simulink model "draft7"  (R2023a)
settings: Solver=VariableStepAuto  StartTime=0.0  StopTime=10  FixedStep=0.0001  MaxStep=0.1  RelTol=1e-3  AbsTol=1e-3  EnableMultiTasking=on
model workspace (MAT data in the model file):
  C_Gimbal = 0.1
  C_IAP = 0.01
  IAP_Pa = 0
  K_Gimbal = 0
  K_IAP = 10
  LeftAbdominalMuscleForce = 0
  LeftBackMuscleForce = 0
  LeftTransverse1MuscleForce = 0
  LeftTransverse2MuscleForce = 0
  Moment_AR = 0
  Moment_FE = 0
  Moment_LB = 0
  RightAbdominalMuscleForce = 0
  RightBackMuscleForce = 0
  RightTransverse1MuscleForce = 0
  RightTransverse2MuscleForce = 0
  a = 1
  b = 1
undefined symbols (not defined in the file): X, Y, Z
libraries: sm_lib x279, nesl_utility x233, simulink_extras x33, checkpacklib x3, simulink x1
(part 6 of 7)

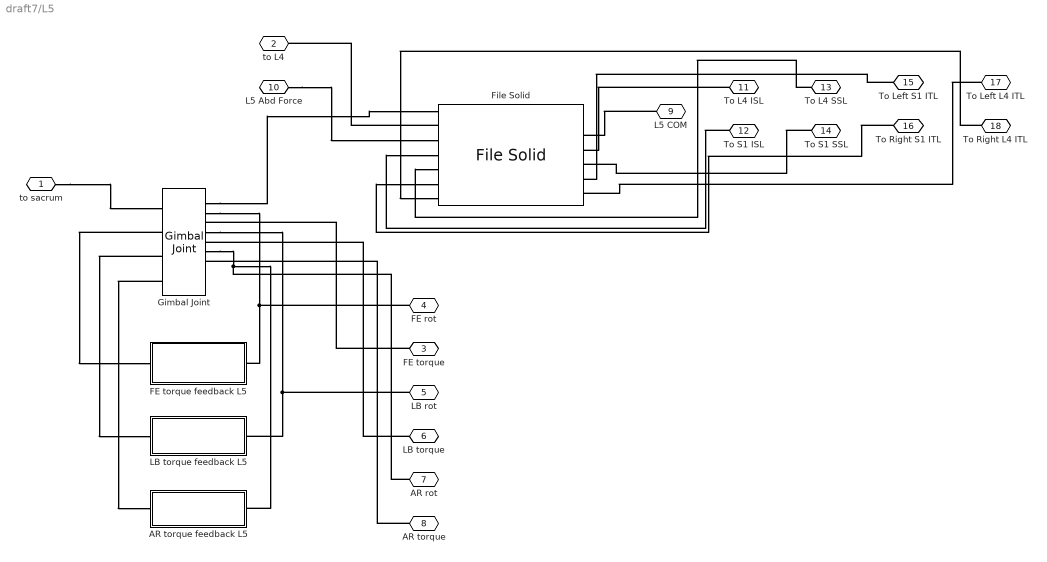
== system draft7/L5 ==
  AR torque feedback L5 : Subsystem
  FE torque feedback L5 : Subsystem
  File Solid : sm_lib/Body Elements/File Solid  ExtGeomFileName=C:\Users\siril\OneDrive\Desktop\TIM-Control\Matlab\Simscape models\CAD - with COM\SymmetricModel\draft7\L5.step  UnitType=FromFile  ExtGeomFileUnits=m  StepReaderType=HEX  ExportConvexHullGeometry=off  InertiaType=CalculateFromGeometry  Mass=1  MassUnits=kg  CenterOfMass=[0 0 0]  CenterOfMassUnits=m  MomentsOfInertia=[1 1 1]  MomentsOfInertiaUnits=kg*m^2  ProductsOfInertia=[0 0 0]  ProductsOfInertiaUnits=kg*m^2  BasedOnType=Density  Density=0.182  DensityUnits=g/cm^3  DoExposeReferenceFrame=on  SerializedFrames=<Frames><Frame><Id>Frame1</Id><Value><Name>To Sacrum</Name><Origin><Source>GeometricFeature</Source><FeatureName>planar surface 1973</FeatureName></Origin><PrimaryAxis><DefinedDirection>+Z</DefinedDirection><Source>GeometricFeature</Source><SourceDirection>+Z</SourceDirection><FeatureName>planar surface 1973</FeatureName></PrimaryAxis><SecondaryAxis><DefinedDirection>+X</DefinedDirection><Source>ReferenceFrame</Source><SourceDirection>+X</SourceDirection><FeatureName></FeatureName></SecondaryAxis></Value></Frame><Frame><Id>Frame2</Id><Value><Name>To L4</Name><Origin><Source>GeometricFeature</Source><FeatureName>planar surface 1977</FeatureName></Origin><PrimaryAxis><DefinedDirection>+Z</DefinedDirection><Source>GeometricFeature</Source><SourceDirection>+Z</SourceDirection><FeatureName>planar surface 1977</FeatureName></PrimaryAxis><SecondaryAxis><DefinedDirection>+X</DefinedDirection><Source>ReferenceFrame</Source><SourceDirection>+X</SourceDirection><FeatureName></FeatureName></SecondaryAxis></Value></Frame><Frame><Id>Frame3</Id><Value><Name>L5 COM</Name><Origin><Source>CenterOfMassFrame</Source><FeatureName></FeatureName></Origin><PrimaryAxis><DefinedDirection>+Z</DefinedDirection><Source>ReferenceFrame</Source><SourceDirection>+Z</SourceDirection><FeatureName></FeatureName></PrimaryAxis><SecondaryAxis><DefinedDirection>+X</DefinedDirection><Source>ReferenceFrame</Source><SourceDirection>+X</SourceDirection><FeatureName></FeatureName></SecondaryAxis></Value></Frame><Frame><Id>Frame4</Id><Value><Name>L5 Abd Force</Name><Origin><Source>GeometricFeature</Source><FeatureName>point 2</FeatureName></Origin><PrimaryAxis><DefinedDirection>+Z</DefinedDirection><Source>GeometricFeature</Source><SourceDirection>+Z</SourceDirection><FeatureName>conical surface 1</FeatureName></PrimaryAxis><SecondaryAxis><DefinedDirection>+X</DefinedDirection><Source>ReferenceFrame</Source><SourceDirection>+X</SourceDirection><FeatureName></FeatureName></SecondaryAxis></Value></Frame><Frame><Id>Frame5</Id><Value><Name>To L4 ISL</Name><Origin><Source>GeometricFeature</Source><FeatureName>point 104</FeatureName></Origin><PrimaryAxis><DefinedDirection>+Z</DefinedDirection><Source>ReferenceFrame</Source><SourceDirection>+Z</SourceDirection><FeatureName></FeatureName></PrimaryAxis><SecondaryAxis><DefinedDirection>+X</DefinedDirection><Source>ReferenceFrame</Source><SourceDirection>+X</SourceDirection><FeatureName></FeatureName></SecondaryAxis></Value></Frame><Frame><Id>Frame6</Id><Value><Name>To S1 ISL</Name><Origin><Source>GeometricFeature</Source><FeatureName>point 11405</FeatureName></Origin><PrimaryAxis><DefinedDirection>+Z</DefinedDirection><Source>ReferenceFrame</Source><SourceDirection>+Z</SourceDirection><FeatureName></FeatureName></PrimaryAxis><SecondaryAxis><DefinedDirection>+X</DefinedDirection><Source>ReferenceFrame</Source><SourceDirection>+X</SourceDirection><FeatureName></FeatureName></SecondaryAxis></Value></Frame><Frame><Id>Frame7</Id><Value><Name>To S1 SSL</Name><Origin><Source>GeometricFeature</Source><FeatureName>point 8728</FeatureName></Origin><PrimaryAxis><DefinedDirection>+Z</DefinedDirection><Source>ReferenceFrame</Source><SourceDirection>+Z</SourceDirection><FeatureName></FeatureName></PrimaryAxis><SecondaryAxis><DefinedDirection>+X</DefinedDirection><Source>ReferenceFrame</Source><SourceDirection>+X</SourceDirection><FeatureName></FeatureName></SecondaryAxis></Value></Frame><Frame><Id>Frame8</Id><Value><Name>To L4 SSL</Name><Origin><Source>GeometricFeature</Source><FeatureName>point 5958</FeatureName></Origin><PrimaryAxis><DefinedDirection>+Z</DefinedDirection><Source>ReferenceFrame</Source><SourceDirection>+Z</SourceDirection><FeatureName></FeatureName></PrimaryAxis><SecondaryAxis><DefinedDirection>+X</DefinedDirection><Source>ReferenceFrame</Source><SourceDirection>+X</SourceDirection><FeatureName></FeatureName></SecondaryAxis></Value></Frame><Frame><Id>Frame9</Id><Value><Name>To Left S1 ITL</Name><Origin><Source>GeometricFeature</Source><FeatureName>point 9071</FeatureName></Origin><PrimaryAxis><DefinedDirection>+Z</DefinedDirection><Source>ReferenceFrame</Source><SourceDirection>+Z</SourceDirection><FeatureName></FeatureName></PrimaryAxis><SecondaryAxis><DefinedDirection>+X</DefinedDirection><Source>ReferenceFrame</Source><SourceDirection>+X</SourceDirection><FeatureName></FeatureName></SecondaryAxis></Value></Frame><Frame><Id>Frame10</Id><Value><Name>To Right S1 ITL</Name><Origin><Source>GeometricFeature</Source><FeatureName>point 3312</FeatureName></Origin><PrimaryAxis><DefinedDirection>+Z</DefinedDirection><Source>ReferenceFrame</Source><SourceDirection>+Z</SourceDirection><FeatureName></FeatureName></PrimaryAxis><SecondaryAxis><DefinedDirection>+X</DefinedDirection><Source>ReferenceFrame</Source><SourceDirection>+X</SourceDirection><FeatureName></FeatureName></SecondaryAxis></Value></Frame><Frame><Id>Frame11</Id><Value><Name>To Left L4 ITL</Name><Origin><Source>GeometricFeature</Source><FeatureName>point 10699</FeatureName></Origin><PrimaryAxis><DefinedDirection>+Z</DefinedDirection><Source>ReferenceFrame</Source><SourceDirection>+Z</SourceDirection><FeatureName></FeatureName></PrimaryAxis><SecondaryAxis><DefinedDirection>+X</DefinedDirection><Source>ReferenceFrame</Source><SourceDirection>+X</SourceDirection><FeatureName></FeatureName></SecondaryAxis></Value></Frame><Frame><Id>Frame12</Id><Value><Name>To Right L4 ITL</Name><Origin><Source>GeometricFeature</Source><FeatureName>point 5014</FeatureName></Origin><PrimaryAxis><DefinedDirection>+Z</DefinedDirection><Source>ReferenceFrame</Source><SourceDirection>+Z</SourceDirection><FeatureName></FeatureName></PrimaryAxis><SecondaryAxis><DefinedDirection>+X</DefinedDirection><Source>ReferenceFrame</Source><SourceDirection>+X</SourceDirection><FeatureName></FeatureName></SecondaryAxis></Value></Frame></Frames>  GraphicType=FromGeometry  MarkerShape=Sphere  MarkerSize=10  GraphicVisPropType=SimpleVisualProperties  GraphicDiffuseColor=[0.5 0.5 0.5]  GraphicSpecularColor=[0.5 0.5 0.5 1.0]  GraphicAmbientColor=[0.15 0.15 0.15 1.0]  GraphicEmissiveColor=[0.0 0.0 0.0 1.0]  GraphicShininess=75  GraphicOpacity=1.0
  Gimbal Joint : sm_lib/Joints/Gimbal Joint  JointMode=Normal  SenseConstraintForce=on  SenseConstraintForceX=off  SenseConstraintForceY=off  SenseConstraintForceZ=off  SenseConstraintTorque=off  SenseConstraintTorqueX=off  SenseConstraintTorqueY=off  SenseConstraintTorqueZ=off  SenseTotalForce=on  SenseTotalForceX=off  SenseTotalForceY=off  SenseTotalForceZ=off  SenseTotalTorque=off  SenseTotalTorqueX=off  SenseTotalTorqueY=off  SenseTotalTorqueZ=off  CompositeWrenchDir=FollowerOnBase  CompositeWrenchFrame=BaseFrame  RxEquilibriumPosition=0  RxEquilibriumPositionUnits=deg  RxSpringStiffness=K_Gimbal  RxSpringStiffnessUnits=N*m/deg  RxDampingCoefficient=C_Gimbal  RxDampingCoefficientUnits=N*m/(deg/s)  RxTorqueActuationMode=InputTorque  RxMotionActuationMode=ComputedMotion  RxSensePosition=on  RxSenseVelocity=off  RxSenseAcceleration=off  RxSenseTorqueForce=on  RxSenseLowerLimitTorqueForce=off  RxSenseUpperLimitTorqueForce=off  RxLowerLimitSpecify=on  RxLowerLimitBound=-30  RxLowerLimitBoundUnits=deg  RxLowerLimitStiffness=10000  RxLowerLimitStiffnessUnits=N*m/deg  RxLowerLimitDamping=100  RxLowerLimitDampingUnits=N*m/(deg/s)  RxLowerLimitTransitionRegionWidth=0.1  RxLowerLimitTransitionRegionWidthUnits=deg  RxUpperLimitSpecify=on  RxUpperLimitBound=30  RxUpperLimitBoundUnits=deg  RxUpperLimitStiffness=10000  RxUpperLimitStiffnessUnits=N*m/deg  RxUpperLimitDamping=100  RxUpperLimitDampingUnits=N*m/(deg/s)  RxUpperLimitTransitionRegionWidth=0.1  RxUpperLimitTransitionRegionWidthUnits=deg  RxPositionTargetSpecify=off  RxPositionTargetPriority=High  RxPositionTargetValue=0  RxPositionTargetValueUnits=deg  RxVelocityTargetSpecify=off  RxVelocityTargetPriority=High  RxVelocityTargetValue=0  RxVelocityTargetValueUnits=deg/s  RyEquilibriumPosition=0  RyEquilibriumPositionUnits=deg  RySpringStiffness=K_Gimbal  RySpringStiffnessUnits=N*m/deg  RyDampingCoefficient=C_Gimbal  RyDampingCoefficientUnits=N*m/(deg/s)  RyTorqueActuationMode=InputTorque  RyMotionActuationMode=ComputedMotion  RySensePosition=on  RySenseVelocity=off  RySenseAcceleration=off  RySenseTorqueForce=on  RySenseLowerLimitTorqueForce=off  RySenseUpperLimitTorqueForce=off  RyLowerLimitSpecify=on  RyLowerLimitBound=-30  RyLowerLimitBoundUnits=deg  RyLowerLimitStiffness=10000  RyLowerLimitStiffnessUnits=N*m/deg  RyLowerLimitDamping=100  RyLowerLimitDampingUnits=N*m/(deg/s)  RyLowerLimitTransitionRegionWidth=0.1  RyLowerLimitTransitionRegionWidthUnits=deg  RyUpperLimitSpecify=on  RyUpperLimitBound=30  RyUpperLimitBoundUnits=deg  RyUpperLimitStiffness=10000  RyUpperLimitStiffnessUnits=N*m/deg  RyUpperLimitDamping=100  RyUpperLimitDampingUnits=N*m/(deg/s)  RyUpperLimitTransitionRegionWidth=0.1  RyUpperLimitTransitionRegionWidthUnits=deg  RyPositionTargetSpecify=off  RyPositionTargetPriority=High  RyPositionTargetValue=0  RyPositionTargetValueUnits=deg  RyVelocityTargetSpecify=off  RyVelocityTargetPriority=High  RyVelocityTargetValue=0  RyVelocityTargetValueUnits=deg/s  RzEquilibriumPosition=0  RzEquilibriumPositionUnits=deg  RzSpringStiffness=K_Gimbal  RzSpringStiffnessUnits=N*m/deg  RzDampingCoefficient=C_Gimbal  RzDampingCoefficientUnits=N*m/(deg/s)  RzTorqueActuationMode=InputTorque  RzMotionActuationMode=ComputedMotion  RzSensePosition=on  RzSenseVelocity=off  RzSenseAcceleration=off  RzSenseTorqueForce=on  RzSenseLowerLimitTorqueForce=off  RzSenseUpperLimitTorqueForce=off  RzLowerLimitSpecify=on  RzLowerLimitBound=-30  RzLowerLimitBoundUnits=deg  RzLowerLimitStiffness=10000  RzLowerLimitStiffnessUnits=N*m/deg  RzLowerLimitDamping=100  RzLowerLimitDampingUnits=N*m/(deg/s)  RzLowerLimitTransitionRegionWidth=0.1  RzLowerLimitTransitionRegionWidthUnits=deg  RzUpperLimitSpecify=on  RzUpperLimitBound=30  RzUpperLimitBoundUnits=deg  RzUpperLimitStiffness=10000  RzUpperLimitStiffnessUnits=N*m/deg  RzUpperLimitDamping=100  RzUpperLimitDampingUnits=N*m/(deg/s)  RzUpperLimitTransitionRegionWidth=0.1  RzUpperLimitTransitionRegionWidthUnits=deg  RzPositionTargetSpecify=off  RzPositionTargetPriority=High  RzPositionTargetValue=0  RzPositionTargetValueUnits=deg  RzVelocityTargetSpecify=off  RzVelocityTargetPriority=High  RzVelocityTargetValue=0  RzVelocityTargetValueUnits=deg/s
  LB torque feedback L5 : Subsystem
  to sacrum : PMIOPort  Side=Left
  to L4 : PMIOPort  Port=2  Side=Right
  FE torque : PMIOPort  Port=3  Side=Right
  FE rot : PMIOPort  Port=4  Side=Right
  LB rot : PMIOPort  Port=5  Side=Right
  LB torque : PMIOPort  Port=6  Side=Right
  AR rot : PMIOPort  Port=7  Side=Right
  AR torque : PMIOPort  Port=8  Side=Right
  L5 COM : PMIOPort  Port=9  Side=Right
  L5 Abd Force : PMIOPort  Port=10  Side=Right
  To L4 ISL : PMIOPort  Port=11  Side=Right
  To S1 ISL : PMIOPort  Port=12  Side=Right
  To L4 SSL : PMIOPort  Port=13  Side=Right
  To S1 SSL : PMIOPort  Port=14  Side=Right
  To Left S1 ITL : PMIOPort  Port=15  Side=Right
  To Right S1 ITL : PMIOPort  Port=16  Side=Right
  To Left L4 ITL : PMIOPort  Port=17  Side=Right
  To Right L4 ITL : PMIOPort  Port=18  Side=Right
  connections:
  File Solid/LConn2 -- to L4/RConn1
  to sacrum/RConn1 -- Gimbal Joint/LConn1
  Gimbal Joint/RConn1 -- File Solid/LConn1
  Gimbal Joint/LConn2 -- FE torque feedback L5/RConn1
  Gimbal Joint/LConn3 -- LB torque feedback L5/RConn1
  Gimbal Joint/LConn4 -- AR torque feedback L5/RConn1
  Gimbal Joint/RConn2 -- FE torque feedback L5/LConn1 -- FE rot/RConn1
  Gimbal Joint/RConn4 -- LB torque feedback L5/LConn1 -- LB rot/RConn1
  Gimbal Joint/RConn6 -- AR rot/RConn1 -- AR torque feedback L5/LConn1
  FE torque/RConn1 -- Gimbal Joint/RConn3
  LB torque/RConn1 -- Gimbal Joint/RConn5
  AR torque/RConn1 -- Gimbal Joint/RConn7
  L5 COM/RConn1 -- File Solid/RConn2
  L5 Abd Force/RConn1 -- File Solid/LConn3
  To L4 ISL/RConn1 -- File Solid/RConn3
  To S1 ISL/RConn1 -- File Solid/LConn4
  To S1 SSL/RConn1 -- File Solid/RConn4
  To L4 SSL/RConn1 -- File Solid/LConn5
  To Left S1 ITL/RConn1 -- File Solid/RConn5
  To Right S1 ITL/RConn1 -- File Solid/LConn6
  To Left L4 ITL/RConn1 -- File Solid/RConn6
  To Right L4 ITL/RConn1 -- File Solid/LConn7

== system draft7/L5-S1 AR ==
  Gain3 : Gain  Gain=-1
  Gain8 : Gain
  L5-S1 AR Simscape : Record  FileSettingsInternal="{\"entries\":[{\"content\":{\"excelSettings\":{\"content\":{},\"type\":\"Streamout.ExcelSettings\"}},\"type\":\"Streamout.FileSettingStorage\",\"uuid\":\"aa947257-96d6-48e4-9108-923ef559b579\"}],\"packageUris\":[\"http://schema.mathworks.com/mf0/streamout_blocks/R2020a\"],\"version\":\"1.0\"}"  Layout=[1 1]  SignalsInternal="{\"entries\":[{\"content\":{\"signals\":[{\"content\":{\"blockPath\":[\"draft7/L5-S1 AR/L5-S1 AR Simscape\"],\"dimensions\":[1],\"domain\":\"draft7/L5-S1 AR/L5-S1 AR Simscape\",\"lineColor\":\"#fe330a\",\"port\":1,\"signalID\":16,\"signalName\":\"L5-S1 AR Simscape Rotation\"},\"type\":\"RecordBlkView.Signal\",\"uuid\":\"ffa9debd-2787-4d27-bfe2-d0c5ad45716a\"},{\"content\":{\"blockPath\":[\"draft7/L5-S1 AR/L5-S1 AR Simscape\"],\"dimensions\":[1],\"domain\":\"draft7/L5-S1 AR/L5-S1 AR Simscape\",\"lineColor\":\"#22b573\",\"port\":2,\"signalID\":19,\"signalName\":\"L5-S1 AR Simscape Moment\"},\"type\":\"RecordBlkView.Signal\",\"uuid\":\"c2a70474-e3ec-479a-a963-718e3afbea8f\"}]},\"type\":\"RecordBlkView.InputSignals\",\"uuid\":\"d6821e1d-03da-4dd5-b040-c2058d2be55c\"}],\"packageUris\":[\"http://schema.mathworks.com/mf0/streamout_blocks/R2020a\"],\"version\":\"1.0\"}"  VisualizationBindings="{\"xyplotplugin\":{\"info\":[{\"series\":[],\"subplotID\":1}]}}"  CompatibilityTag=XY
  PS-Simulink Converter : nesl_utility/PS-Simulink Converter  PhysicalDomain=network_engine_domain  SubClassName=ps_output  LeftPortType=input  RightPortType=output  PseudoPeriodic=off  Frequencies=[]  VectorFormat=1-D array  Unit=rad  AffineConversion=off
  PS-Simulink Converter7 : nesl_utility/PS-Simulink Converter  PhysicalDomain=network_engine_domain  SubClassName=ps_output  LeftPortType=input  RightPortType=output  PseudoPeriodic=off  Frequencies=[]  VectorFormat=1-D array  Unit=N*m  AffineConversion=off
  Radians to Degrees : simulink_extras/Transformations/Radians to Degrees
  Scope10 : Scope
  Scope11 : Scope
  Moment : PMIOPort  Side=Left
  Rotation : PMIOPort  Port=2  Side=Left
  wires:
  Radians to Degrees/1 -> Gain3/1
  Gain8/1 -> L5-S1 AR Simscape/2, Scope11/1  "L5-S1 AR Simscape Moment"
  Gain3/1 -> L5-S1 AR Simscape/1, Scope10/1  "L5-S1 AR Simscape Rotation"
  PS-Simulink Converter/1 -> Radians to Degrees/1
  PS-Simulink Converter7/1 -> Gain8/1
  connections:
  Rotation/RConn1 -- PS-Simulink Converter/LConn1
  Moment/RConn1 -- PS-Simulink Converter7/LConn1

== system draft7/L5-S1 FE ==
  Gain3 : Gain  Gain=-1
  Gain8 : Gain
  L5-S1 FE Simscape : Record  FileSettingsInternal="{\"entries\":[{\"content\":{\"excelSettings\":{\"content\":{},\"type\":\"Streamout.ExcelSettings\"}},\"type\":\"Streamout.FileSettingStorage\",\"uuid\":\"151b2801-b1d4-4853-8f15-4c7b111b7120\"}],\"packageUris\":[\"http://schema.mathworks.com/mf0/streamout_blocks/R2020a\"],\"version\":\"1.0\"}"  Layout=[1 1]  SignalsInternal="{\"entries\":[{\"content\":{\"signals\":[{\"content\":{\"blockPath\":[\"draft7/L5-S1 FE/L5-S1 FE Simscape\"],\"dimensions\":[1],\"domain\":\"draft7/L5-S1 FE/L5-S1 FE Simscape\",\"lineColor\":\"#0072bd\",\"port\":1,\"signalID\":72,\"signalName\":\"L5-S1 FE Simscape Rotation\"},\"type\":\"RecordBlkView.Signal\",\"uuid\":\"2f8118ae-f7f6-41cc-b921-4eddef1adc90\"},{\"content\":{\"blockPath\":[\"draft7/L5-S1 FE/L5-S1 FE Simscape\"],\"dimensions\":[1],\"domain\":\"draft7/L5-S1 FE/L5-S1 FE Simscape\",\"lineColor\":\"#d95319\",\"port\":2,\"signalID\":75,\"signalName\":\"L5-S1 FE Simscape Moment\"},\"type\":\"RecordBlkView.Signal\",\"uuid\":\"d142d7e5-5d32-45b6-99aa-7d1bd87efb45\"}]},\"type\":\"RecordBlkView.InputSignals\",\"uuid\":\"516e9dee-34af-4479-a0ea-4dee4e67571b\"}],\"packageUris\":[\"http://schema.mathworks.com/mf0/streamout_blocks/R2020a\"],\"version\":\"1.0\"}"  VisualizationBindings="{\"xyplotplugin\":{\"info\":[{\"series\":[],\"subplotID\":1}]}}"  CompatibilityTag=XY
  PS-Simulink Converter : nesl_utility/PS-Simulink Converter  PhysicalDomain=network_engine_domain  SubClassName=ps_output  LeftPortType=input  RightPortType=output  PseudoPeriodic=off  Frequencies=[]  VectorFormat=1-D array  Unit=rad  AffineConversion=off
  PS-Simulink Converter7 : nesl_utility/PS-Simulink Converter  PhysicalDomain=network_engine_domain  SubClassName=ps_output  LeftPortType=input  RightPortType=output  PseudoPeriodic=off  Frequencies=[]  VectorFormat=1-D array  Unit=N*m  AffineConversion=off
  Radians to Degrees : simulink_extras/Transformations/Radians to Degrees
  Scope10 : Scope
  Scope11 : Scope
  Moment : PMIOPort  Side=Left
  Rotation : PMIOPort  Port=2  Side=Left
  wires:
  Radians to Degrees/1 -> Gain3/1
  Gain8/1 -> L5-S1 FE Simscape/2, Scope11/1  "L5-S1 FE Simscape Moment"
  Gain3/1 -> L5-S1 FE Simscape/1, Scope10/1  "L5-S1 FE Simscape Rotation"
  PS-Simulink Converter/1 -> Radians to Degrees/1
  PS-Simulink Converter7/1 -> Gain8/1
  connections:
  Rotation/RConn1 -- PS-Simulink Converter/LConn1
  Moment/RConn1 -- PS-Simulink Converter7/LConn1

== system draft7/L5-S1 LB ==
  Gain3 : Gain
  Gain8 : Gain  Gain=-1
  L5-S1 LB Simscape : Record  FileSettingsInternal="{\"entries\":[{\"content\":{\"excelSettings\":{\"content\":{},\"type\":\"Streamout.ExcelSettings\"}},\"type\":\"Streamout.FileSettingStorage\",\"uuid\":\"005a565d-736e-4536-9ba4-b6b5e310d41f\"}],\"packageUris\":[\"http://schema.mathworks.com/mf0/streamout_blocks/R2020a\"],\"version\":\"1.0\"}"  Layout=[1 1]  SignalsInternal="{\"entries\":[{\"content\":{\"signals\":[{\"content\":{\"blockPath\":[\"draft7/L5-S1 LB/L5-S1 LB Simscape\"],\"dimensions\":[1],\"domain\":\"draft7/L5-S1 LB/L5-S1 LB Simscape\",\"lineColor\":\"#edb120\",\"port\":1,\"signalID\":8,\"signalName\":\"L5-S1 LB Simscape Rotation\"},\"type\":\"RecordBlkView.Signal\",\"uuid\":\"56eef16f-aea4-4a9c-b47a-1242a6e60a09\"},{\"content\":{\"blockPath\":[\"draft7/L5-S1 LB/L5-S1 LB Simscape\"],\"dimensions\":[1],\"domain\":\"draft7/L5-S1 LB/L5-S1 LB Simscape\",\"lineColor\":\"#7e2f8e\",\"port\":2,\"signalID\":11,\"signalName\":\"L5-S1 LB Simscape Moment\"},\"type\":\"RecordBlkView.Signal\",\"uuid\":\"bc9889e2-1c41-435c-b871-624510f5e24b\"}]},\"type\":\"RecordBlkView.InputSignals\",\"uuid\":\"6c571820-3a7e-4cad-af8a-f14e824932b2\"}],\"packageUris\":[\"http://schema.mathworks.com/mf0/streamout_blocks/R2020a\"],\"version\":\"1.0\"}"  VisualizationBindings="{\"xyplotplugin\":{\"info\":[{\"series\":[],\"subplotID\":1}]}}"  CompatibilityTag=XY
  PS-Simulink Converter : nesl_utility/PS-Simulink Converter  PhysicalDomain=network_engine_domain  SubClassName=ps_output  LeftPortType=input  RightPortType=output  PseudoPeriodic=off  Frequencies=[]  VectorFormat=1-D array  Unit=rad  AffineConversion=off
  PS-Simulink Converter7 : nesl_utility/PS-Simulink Converter  PhysicalDomain=network_engine_domain  SubClassName=ps_output  LeftPortType=input  RightPortType=output  PseudoPeriodic=off  Frequencies=[]  VectorFormat=1-D array  Unit=N*m  AffineConversion=off
  Radians to Degrees : simulink_extras/Transformations/Radians to Degrees
  Scope10 : Scope
  Scope11 : Scope
  Moment : PMIOPort  Side=Left
  Rotation : PMIOPort  Port=2  Side=Left
  wires:
  Radians to Degrees/1 -> Gain3/1
  Gain8/1 -> L5-S1 LB Simscape/2, Scope11/1  "L5-S1 LB Simscape Moment"
  Gain3/1 -> L5-S1 LB Simscape/1, Scope10/1  "L5-S1 LB Simscape Rotation"
  PS-Simulink Converter/1 -> Radians to Degrees/1
  PS-Simulink Converter7/1 -> Gain8/1
  connections:
  Rotation/RConn1 -- PS-Simulink Converter/LConn1
  Moment/RConn1 -- PS-Simulink Converter7/LConn1

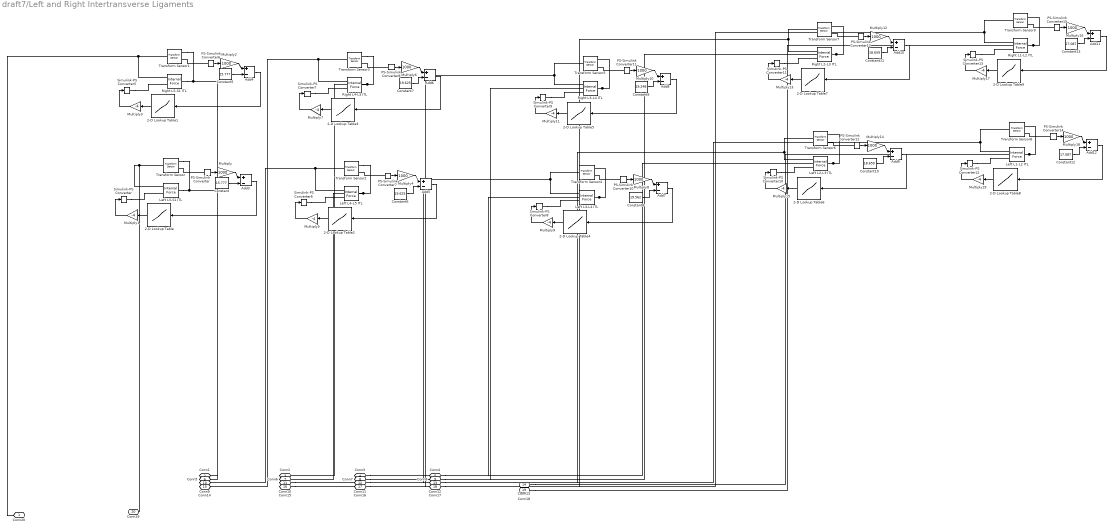
== system draft7/Left and Right Intertransverse Ligaments ==
  2-D Lookup Table : Lookup_n-D  NumberOfTableDimensions=1  BreakpointsForDimension1=[0;0.178;2.67;3.916;5.34]  BreakpointsForDimension2=[1:3]  Table=[0;0;3;7.5;30]  InternalRulePriority=Speed  RndMeth=Simplest
  2-D Lookup Table1 : Lookup_n-D  NumberOfTableDimensions=1  BreakpointsForDimension1=[0;0.178;2.67;3.916;5.34]  BreakpointsForDimension2=[1:3]  Table=[0;0;3;7.5;30]  InternalRulePriority=Speed  RndMeth=Simplest
  2-D Lookup Table2 : Lookup_n-D  NumberOfTableDimensions=1  BreakpointsForDimension1=[0;0.213;3.195;4.686;6.39]  BreakpointsForDimension2=[1:3]  Table=[0;0;3;7.5;30]  InternalRulePriority=Speed  RndMeth=Simplest
  2-D Lookup Table3 : Lookup_n-D  NumberOfTableDimensions=1  BreakpointsForDimension1=[0;0.213;3.195;4.686;6.39]  BreakpointsForDimension2=[1:3]  Table=[0;0;3;7.5;30]  InternalRulePriority=Speed  RndMeth=Simplest
  2-D Lookup Table4 : Lookup_n-D  NumberOfTableDimensions=1  BreakpointsForDimension1=[0;0.1985;2.9775;4.367;5.955]  BreakpointsForDimension2=[1:3]  Table=[0;0;3;7.5;30]  InternalRulePriority=Speed  RndMeth=Simplest
  2-D Lookup Table5 : Lookup_n-D  NumberOfTableDimensions=1  BreakpointsForDimension1=[0;0.1985;2.9775;4.367;5.955]  BreakpointsForDimension2=[1:3]  Table=[0;0;3;7.5;30]  InternalRulePriority=Speed  RndMeth=Simplest
  2-D Lookup Table6 : Lookup_n-D  NumberOfTableDimensions=1  BreakpointsForDimension1=[0;0.2084;3.126;4.5848;6.252]  BreakpointsForDimension2=[1:3]  Table=[0;0;3;7.5;30]  InternalRulePriority=Speed  RndMeth=Simplest
  2-D Lookup Table7 : Lookup_n-D  NumberOfTableDimensions=1  BreakpointsForDimension1=[0;0.2084;3.126;4.5848;6.252]  BreakpointsForDimension2=[1:3]  Table=[0;0;3;7.5;30]  InternalRulePriority=Speed  RndMeth=Simplest
  2-D Lookup Table8 : Lookup_n-D  NumberOfTableDimensions=1  BreakpointsForDimension1=[0;0.1966;2.949;4.3252;5.898]  BreakpointsForDimension2=[1:3]  Table=[0;0;3;7.5;30]  InternalRulePriority=Speed  RndMeth=Simplest
  2-D Lookup Table9 : Lookup_n-D  NumberOfTableDimensions=1  BreakpointsForDimension1=[0;0.1966;2.949;4.3252;5.898]  BreakpointsForDimension2=[1:3]  Table=[0;0;3;7.5;30]  InternalRulePriority=Speed  RndMeth=Simplest
  Add{3..12} (10 alike) : Sum  Inputs=+-
  Constant : Constant  Value=15.777
  Constant10 : Constant  Value=18.659
  Constant11 : Constant  Value=18.659
  Constant12 : Constant  Value=17.087
  Constant13 : Constant  Value=17.087
  Constant5 : Constant  Value=15.777
  Constant6 : Constant  Value=19.625
  Constant7 : Constant  Value=19.625
  Constant8 : Constant  Value=19.562
  Constant9 : Constant  Value=19.248
  Left L1-L2 ITL : sm_lib/Forces and Torques/Internal Force
  Left L2-L3 ITL : sm_lib/Forces and Torques/Internal Force
  Left L3-L4 ITL : sm_lib/Forces and Torques/Internal Force
  Left L4-L5 ITL : sm_lib/Forces and Torques/Internal Force
  Left L5-S1 ITL : sm_lib/Forces and Torques/Internal Force
  Multiply{,2,4,6,8,10,12,14,16,18} (10 alike) : Gain  Gain=1000
  Multiply{1,3,5,7,9,11,13,15,17,19} (10 alike) : Gain  Gain=-4
  PS-Simulink Converter{,6..8,10..15} (10 alike) : nesl_utility/PS-Simulink Converter  PhysicalDomain=network_engine_domain  SubClassName=ps_output  LeftPortType=input  RightPortType=output  PseudoPeriodic=off  Frequencies=[]  VectorFormat=inherit  Unit=inherit  AffineConversion=off
  Right L1-L2 ITL : sm_lib/Forces and Torques/Internal Force
  Right L2-L3 ITL : sm_lib/Forces and Torques/Internal Force
  Right L3-L4 ITL : sm_lib/Forces and Torques/Internal Force
  Right L4-L5 ITL : sm_lib/Forces and Torques/Internal Force
  Right L5-S1 ITL : sm_lib/Forces and Torques/Internal Force
  Simulink-PS Converter{,5..13} (10 alike) : nesl_utility/Simulink-PS Converter  PhysicalDomain=network_engine_domain  SubClassName=ps_input  LeftPortType=input  RightPortType=output  PseudoPeriodic=off  Frequencies=[]  NoiseDistribution=none  NoiseParameters=[]  Unit=1  AffineConversion=off  FilteringAndDerivatives=provide  SimscapeFilterOrder=1  InputFilterTimeConstant=0.001  UdotUserProvided=0
  Transform Sensor{,1..9} (10 alike) : sm_lib/Frames and Transforms/Transform Sensor  MeasurementFrame=World  RotationSequence=XYX  SenseAngle=off  SenseAxis=off  SenseQ=off  SenseR=off  SenseRotationSequence=off  SenseOmegaX=off  SenseOmegaY=off  SenseOmegaZ=off  SenseQDot=off  SenseRDot=off  SenseRotationSequenceDot=off  SenseAlphaX=off  SenseAlphaY=off  SenseAlphaZ=off  SenseQDDot=off  SenseRDDot=off  SenseX=off  SenseY=off  SenseZ=off  SenseRad=off  SenseAzim=off  SenseDist=on  SenseInc=off  SenseXDot=off  SenseYDot=off  SenseZDot=off  SenseRadDot=off  SenseAzimDot=off  SenseDistDot=off  SenseIncDot=off  SenseXDDot=off  SenseYDDot=off  SenseZDDot=off  SenseRadDDot=off  SenseAzimDDot=off  SenseDistDDot=off  SenseIncDDot=off
  Conn20 : PMIOPort  Side=Left
  Conn1 : PMIOPort  Port=2  Side=Left
  Conn2 : PMIOPort  Port=3  Side=Left
  Conn3 : PMIOPort  Port=4  Side=Left
  Conn4 : PMIOPort  Port=5  Side=Left
  Conn5 : PMIOPort  Port=6  Side=Left
  Conn6 : PMIOPort  Port=7  Side=Left
  Conn7 : PMIOPort  Port=8  Side=Left
  Conn8 : PMIOPort  Port=9  Side=Left
  Conn9 : PMIOPort  Port=10  Side=Left
  Conn10 : PMIOPort  Port=11  Side=Left
  Conn11 : PMIOPort  Port=12  Side=Left
  Conn12 : PMIOPort  Port=13  Side=Left
  Conn13 : PMIOPort  Port=14  Side=Left
  Conn14 : PMIOPort  Port=15  Side=Left
  Conn15 : PMIOPort  Port=16  Side=Left
  Conn16 : PMIOPort  Port=17  Side=Left
  Conn17 : PMIOPort  Port=18  Side=Left
  Conn18 : PMIOPort  Port=19  Side=Left
  Conn19 : PMIOPort  Port=20  Side=Left
  wires:
  Multiply18/1 -> Add12/1
  Add8/1 -> 2-D Lookup Table5/1
  Add12/1 -> 2-D Lookup Table8/1
  Constant6/1 -> Add5/2
  Constant9/1 -> Add8/2
  Add5/1 -> 2-D Lookup Table2/1
  Multiply16/1 -> Add11/1
  2-D Lookup Table/1 -> Multiply1/1
  Multiply17/1 -> Simulink-PS Converter13/1
  Add6/1 -> 2-D Lookup Table3/1
  Constant11/1 -> Add10/2
  2-D Lookup Table9/1 -> Multiply17/1
  2-D Lookup Table8/1 -> Multiply19/1
  Multiply7/1 -> Simulink-PS Converter7/1
  2-D Lookup Table3/1 -> Multiply7/1
  PS-Simulink Converter8/1 -> Multiply6/1
  Multiply6/1 -> Add6/1
  PS-Simulink Converter7/1 -> Multiply4/1
  Multiply5/1 -> Simulink-PS Converter6/1
  Constant12/1 -> Add12/2
  Constant8/1 -> Add7/2
  Constant7/1 -> Add6/2
  Multiply14/1 -> Add9/1
  Multiply8/1 -> Add7/1
  2-D Lookup Table2/1 -> Multiply5/1
  Multiply4/1 -> Add5/1
  Add7/1 -> 2-D Lookup Table4/1
  Multiply19/1 -> Simulink-PS Converter12/1
  PS-Simulink Converter15/1 -> Multiply16/1
  Add11/1 -> 2-D Lookup Table9/1
  Constant13/1 -> Add11/2
  PS-Simulink Converter10/1 -> Multiply8/1
  PS-Simulink Converter14/1 -> Multiply18/1
  2-D Lookup Table4/1 -> Multiply9/1
  Multiply9/1 -> Simulink-PS Converter8/1
  PS-Simulink Converter11/1 -> Multiply10/1
  Multiply10/1 -> Add8/1
  Multiply11/1 -> Simulink-PS Converter9/1
  2-D Lookup Table5/1 -> Multiply11/1
  PS-Simulink Converter12/1 -> Multiply14/1
  Add9/1 -> 2-D Lookup Table6/1
  Constant10/1 -> Add9/2
  Add10/1 -> 2-D Lookup Table7/1
  2-D Lookup Table6/1 -> Multiply15/1
  Constant/1 -> Add3/2
  Multiply1/1 -> Simulink-PS Converter/1
  Multiply/1 -> Add3/1
  2-D Lookup Table7/1 -> Multiply13/1
  Add3/1 -> 2-D Lookup Table/1
  PS-Simulink Converter/1 -> Multiply/1
  Multiply15/1 -> Simulink-PS Converter10/1
  PS-Simulink Converter13/1 -> Multiply12/1
  Multiply12/1 -> Add10/1
  Multiply13/1 -> Simulink-PS Converter11/1
  Constant5/1 -> Add4/2
  Add4/1 -> 2-D Lookup Table1/1
  2-D Lookup Table1/1 -> Multiply3/1
  Multiply2/1 -> Add4/1
  PS-Simulink Converter6/1 -> Multiply2/1
  Multiply3/1 -> Simulink-PS Converter5/1
  connections:
  Right L2-L3 ITL/RConn1 -- Transform Sensor7/RConn1 -- Conn8/RConn1
  Transform Sensor7/LConn1 -- Conn16/RConn1 -- Right L2-L3 ITL/LConn1
  Transform Sensor6/LConn1 -- Conn11/RConn1 -- Left L2-L3 ITL/LConn1
  Right L1-L2 ITL/RConn1 -- Transform Sensor9/RConn1 -- Conn18/RConn1
  Left L4-L5 ITL/RConn1 -- Transform Sensor2/RConn1 -- Conn6/RConn1
  Simulink-PS Converter12/RConn1 -- Left L1-L2 ITL/LConn2
  Right L3-L4 ITL/RConn1 -- Transform Sensor5/RConn1 -- Conn7/RConn1
  Left L2-L3 ITL/RConn1 -- Transform Sensor6/RConn1 -- Conn4/RConn1
  Simulink-PS Converter11/RConn1 -- Right L2-L3 ITL/LConn2
  Simulink-PS Converter6/RConn1 -- Left L4-L5 ITL/LConn2
  PS-Simulink Converter13/LConn1 -- Transform Sensor7/RConn2
  Simulink-PS Converter10/RConn1 -- Left L2-L3 ITL/LConn2
  Left L5-S1 ITL/RConn1 -- Conn1/RConn1 -- Transform Sensor/RConn1
  Left L1-L2 ITL/RConn1 -- Transform Sensor8/RConn1 -- Conn13/RConn1
  Simulink-PS Converter7/RConn1 -- Right L4-L5 ITL/LConn2
  Transform Sensor8/LConn1 -- Conn12/RConn1 -- Left L1-L2 ITL/LConn1
  Transform Sensor4/LConn1 -- Conn10/RConn1 -- Left L3-L4 ITL/LConn1
  Simulink-PS Converter8/RConn1 -- Left L3-L4 ITL/LConn2
  PS-Simulink Converter7/LConn1 -- Transform Sensor2/RConn2
  Transform Sensor3/LConn1 -- Conn14/RConn1 -- Right L4-L5 ITL/LConn1
  PS-Simulink Converter8/LConn1 -- Transform Sensor3/RConn2
  Transform Sensor9/LConn1 -- Conn17/RConn1 -- Right L1-L2 ITL/LConn1
  Transform Sensor2/LConn1 -- Conn9/RConn1 -- Left L4-L5 ITL/LConn1
  PS-Simulink Converter10/LConn1 -- Transform Sensor4/RConn2
  Right L4-L5 ITL/RConn1 -- Transform Sensor3/RConn1 -- Conn2/RConn1
  PS-Simulink Converter15/LConn1 -- Transform Sensor9/RConn2
  Simulink-PS Converter5/RConn1 -- Right L5-S1 ITL/LConn2
  Left L3-L4 ITL/RConn1 -- Transform Sensor4/RConn1 -- Conn3/RConn1
  Simulink-PS Converter13/RConn1 -- Right L1-L2 ITL/LConn2
  PS-Simulink Converter14/LConn1 -- Transform Sensor8/RConn2
  Simulink-PS Converter9/RConn1 -- Right L3-L4 ITL/LConn2
  PS-Simulink Converter11/LConn1 -- Transform Sensor5/RConn2
  Transform Sensor5/LConn1 -- Conn15/RConn1 -- Right L3-L4 ITL/LConn1
  Left L5-S1 ITL/LConn1 -- Transform Sensor/LConn1 -- Conn19/RConn1
  PS-Simulink Converter/LConn1 -- Transform Sensor/RConn2
  Simulink-PS Converter/RConn1 -- Left L5-S1 ITL/LConn2
  PS-Simulink Converter12/LConn1 -- Transform Sensor6/RConn2
  Right L5-S1 ITL/RConn1 -- Conn5/RConn1 -- Transform Sensor1/RConn1
  Transform Sensor1/LConn1 -- Conn20/RConn1 -- Right L5-S1 ITL/LConn1
  PS-Simulink Converter6/LConn1 -- Transform Sensor1/RConn2

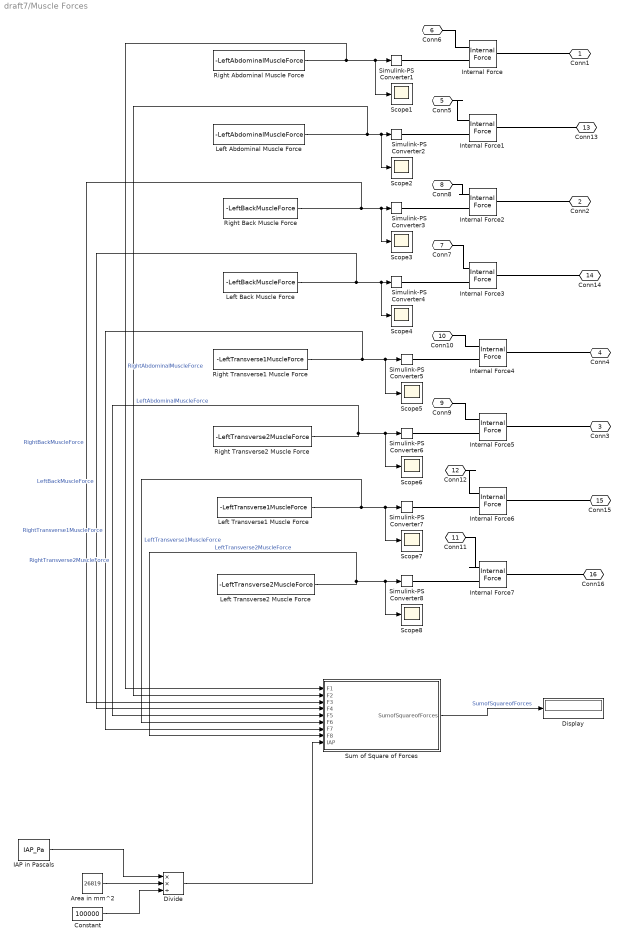
== system draft7/Muscle Forces ==
  Area in mm^2 : Constant  Value=26819
  Constant : Constant  Value=100000
  Display : Display
  Divide : Product  Inputs=**/
  IAP in Pascals : Constant  Value=IAP_Pa
  Internal Force{,1..7} (8 alike) : sm_lib/Forces and Torques/Internal Force
  Left Abdominal Muscle Force : Constant  Value=-LeftAbdominalMuscleForce
  Left Back Muscle Force : Constant  Value=-LeftBackMuscleForce
  Left Transverse1 Muscle Force : Constant  Value=-LeftTransverse1MuscleForce
  Left Transverse2 Muscle Force : Constant  Value=-LeftTransverse2MuscleForce
  Right Abdominal Muscle Force : Constant  Value=-LeftAbdominalMuscleForce
  Right Back Muscle Force : Constant  Value=-LeftBackMuscleForce
  Right Transverse1 Muscle Force : Constant  Value=-LeftTransverse1MuscleForce
  Right Transverse2 Muscle Force : Constant  Value=-LeftTransverse2MuscleForce
  Scope{1..8} (8 alike) : Scope
  Simulink-PS Converter{1..8} (8 alike) : nesl_utility/Simulink-PS Converter  PhysicalDomain=network_engine_domain  SubClassName=ps_input  LeftPortType=input  RightPortType=output  PseudoPeriodic=off  Frequencies=[]  NoiseDistribution=none  NoiseParameters=[]  Unit=1  AffineConversion=off  FilteringAndDerivatives=provide  SimscapeFilterOrder=1  InputFilterTimeConstant=0.001  UdotUserProvided=0
  Sum of Square of Forces : MATLAB Function  TreatAsAtomicUnit=on
  Conn1 : PMIOPort  Side=Right
  Conn2 : PMIOPort  Port=2  Side=Right
  Conn3 : PMIOPort  Port=3  Side=Right
  Conn4 : PMIOPort  Port=4  Side=Right
  Conn5 : PMIOPort  Port=5  Side=Left
  Conn6 : PMIOPort  Port=6  Side=Left
  Conn7 : PMIOPort  Port=7  Side=Left
  Conn8 : PMIOPort  Port=8  Side=Left
  Conn9 : PMIOPort  Port=9  Side=Left
  Conn10 : PMIOPort  Port=10  Side=Left
  Conn11 : PMIOPort  Port=11  Side=Left
  Conn12 : PMIOPort  Port=12  Side=Left
  Conn13 : PMIOPort  Port=13  Side=Right
  Conn14 : PMIOPort  Port=14  Side=Right
  Conn15 : PMIOPort  Port=15  Side=Right
  Conn16 : PMIOPort  Port=16  Side=Right
  wires:
  Sum of Square of Forces/1(SumofSquareofForces) -> Display/1  "SumofSquareofForces"
  Right Abdominal Muscle Force/1 -> Scope1/1, Simulink-PS Converter1/1, Sum of Square of Forces/1(F1)  "RightAbdominalMuscleForce"
  Left Abdominal Muscle Force/1 -> Scope2/1, Simulink-PS Converter2/1, Sum of Square of Forces/2(F2)  "LeftAbdominalMuscleForce"
  Right Back Muscle Force/1 -> Scope3/1, Simulink-PS Converter3/1, Sum of Square of Forces/3(F3)  "RightBackMuscleForce"
  Left Back Muscle Force/1 -> Sum of Square of Forces/4(F4), Scope4/1, Simulink-PS Converter4/1  "LeftBackMuscleForce"
  Right Transverse2 Muscle Force/1 -> Sum of Square of Forces/5(F5), Scope6/1, Simulink-PS Converter6/1  "RightTransverse2MuscleForce"
  Left Transverse1 Muscle Force/1 -> Scope7/1, Simulink-PS Converter7/1, Sum of Square of Forces/6(F6)  "LeftTransverse1MuscleForce"
  Right Transverse1 Muscle Force/1 -> Scope5/1, Simulink-PS Converter5/1, Sum of Square of Forces/7(F7)  "RightTransverse1MuscleForce"
  Left Transverse2 Muscle Force/1 -> Sum of Square of Forces/8(F8), Scope8/1, Simulink-PS Converter8/1  "LeftTransverse2MuscleForce"
  IAP in Pascals/1 -> Divide/1
  Constant/1 -> Divide/3
  Area in mm^2/1 -> Divide/2
  Divide/1 -> Sum of Square of Forces/9(IAP)
  connections:
  Internal Force2/LConn1 -- Conn8/RConn1
  Conn7/RConn1 -- Internal Force3/LConn1
  Simulink-PS Converter8/RConn1 -- Internal Force7/LConn2
  Conn4/RConn1 -- Internal Force4/RConn1
  Simulink-PS Converter6/RConn1 -- Internal Force5/LConn2
  Simulink-PS Converter1/RConn1 -- Internal Force/LConn2
  Conn15/RConn1 -- Internal Force6/RConn1
  Conn3/RConn1 -- Internal Force5/RConn1
  Internal Force7/LConn1 -- Conn11/RConn1
  Conn2/RConn1 -- Internal Force2/RConn1
  Conn13/RConn1 -- Internal Force1/RConn1
  Conn1/RConn1 -- Internal Force/RConn1
  Simulink-PS Converter2/RConn1 -- Internal Force1/LConn2
  Simulink-PS Converter3/RConn1 -- Internal Force2/LConn2
  Conn6/RConn1 -- Internal Force/LConn1
  Simulink-PS Converter4/RConn1 -- Internal Force3/LConn2
  Simulink-PS Converter5/RConn1 -- Internal Force4/LConn2
  Simulink-PS Converter7/RConn1 -- Internal Force6/LConn2
  Conn14/RConn1 -- Internal Force3/RConn1
  Conn9/RConn1 -- Internal Force5/LConn1
  Conn10/RConn1 -- Internal Force4/LConn1
  Conn12/RConn1 -- Internal Force6/LConn1
  Conn16/RConn1 -- Internal Force7/RConn1
  Conn5/RConn1 -- Internal Force1/LConn1

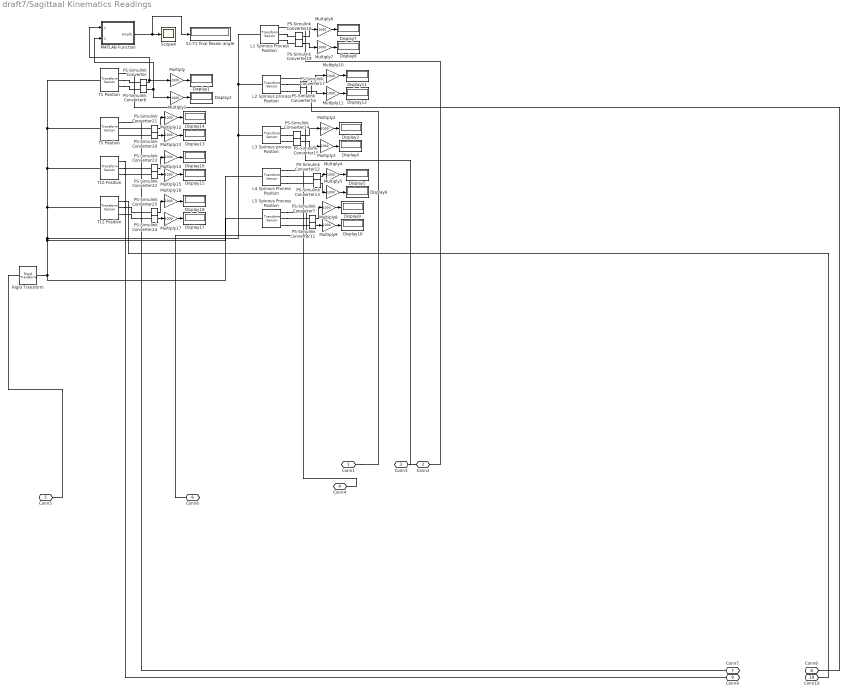
== system draft7/Sagittaal Kinematics Readings ==
  Display{1..18} (18 alike) : Display
  L1 Spinous Process Position : sm_lib/Frames and Transforms/Transform Sensor  MeasurementFrame=World  RotationSequence=XYX  SenseAngle=off  SenseAxis=off  SenseQ=off  SenseR=off  SenseRotationSequence=off  SenseOmegaX=off  SenseOmegaY=off  SenseOmegaZ=off  SenseQDot=off  SenseRDot=off  SenseRotationSequenceDot=off  SenseAlphaX=off  SenseAlphaY=off  SenseAlphaZ=off  SenseQDDot=off  SenseRDDot=off  SenseX=off  SenseY=on  SenseZ=on  SenseRad=off  SenseAzim=off  SenseDist=off  SenseInc=off  SenseXDot=off  SenseYDot=off  SenseZDot=off  SenseRadDot=off  SenseAzimDot=off  SenseDistDot=off  SenseIncDot=off  SenseXDDot=off  SenseYDDot=off  SenseZDDot=off  SenseRadDDot=off  SenseAzimDDot=off  SenseDistDDot=off  SenseIncDDot=off
  L2 Spinous process Position : sm_lib/Frames and Transforms/Transform Sensor  MeasurementFrame=World  RotationSequence=XYX  SenseAngle=off  SenseAxis=off  SenseQ=off  SenseR=off  SenseRotationSequence=off  SenseOmegaX=off  SenseOmegaY=off  SenseOmegaZ=off  SenseQDot=off  SenseRDot=off  SenseRotationSequenceDot=off  SenseAlphaX=off  SenseAlphaY=off  SenseAlphaZ=off  SenseQDDot=off  SenseRDDot=off  SenseX=off  SenseY=on  SenseZ=on  SenseRad=off  SenseAzim=off  SenseDist=off  SenseInc=off  SenseXDot=off  SenseYDot=off  SenseZDot=off  SenseRadDot=off  SenseAzimDot=off  SenseDistDot=off  SenseIncDot=off  SenseXDDot=off  SenseYDDot=off  SenseZDDot=off  SenseRadDDot=off  SenseAzimDDot=off  SenseDistDDot=off  SenseIncDDot=off
  L3 Spinous process Position : sm_lib/Frames and Transforms/Transform Sensor  MeasurementFrame=World  RotationSequence=XYX  SenseAngle=off  SenseAxis=off  SenseQ=off  SenseR=off  SenseRotationSequence=off  SenseOmegaX=off  SenseOmegaY=off  SenseOmegaZ=off  SenseQDot=off  SenseRDot=off  SenseRotationSequenceDot=off  SenseAlphaX=off  SenseAlphaY=off  SenseAlphaZ=off  SenseQDDot=off  SenseRDDot=off  SenseX=off  SenseY=on  SenseZ=on  SenseRad=off  SenseAzim=off  SenseDist=off  SenseInc=off  SenseXDot=off  SenseYDot=off  SenseZDot=off  SenseRadDot=off  SenseAzimDot=off  SenseDistDot=off  SenseIncDot=off  SenseXDDot=off  SenseYDDot=off  SenseZDDot=off  SenseRadDDot=off  SenseAzimDDot=off  SenseDistDDot=off  SenseIncDDot=off
  L4 Spinous Process Position : sm_lib/Frames and Transforms/Transform Sensor  MeasurementFrame=World  RotationSequence=XYX  SenseAngle=off  SenseAxis=off  SenseQ=off  SenseR=off  SenseRotationSequence=off  SenseOmegaX=off  SenseOmegaY=off  SenseOmegaZ=off  SenseQDot=off  SenseRDot=off  SenseRotationSequenceDot=off  SenseAlphaX=off  SenseAlphaY=off  SenseAlphaZ=off  SenseQDDot=off  SenseRDDot=off  SenseX=off  SenseY=on  SenseZ=on  SenseRad=off  SenseAzim=off  SenseDist=off  SenseInc=off  SenseXDot=off  SenseYDot=off  SenseZDot=off  SenseRadDot=off  SenseAzimDot=off  SenseDistDot=off  SenseIncDot=off  SenseXDDot=off  SenseYDDot=off  SenseZDDot=off  SenseRadDDot=off  SenseAzimDDot=off  SenseDistDDot=off  SenseIncDDot=off
  L5 Spinous Process Position : sm_lib/Frames and Transforms/Transform Sensor  MeasurementFrame=World  RotationSequence=XYX  SenseAngle=off  SenseAxis=off  SenseQ=off  SenseR=off  SenseRotationSequence=off  SenseOmegaX=off  SenseOmegaY=off  SenseOmegaZ=off  SenseQDot=off  SenseRDot=off  SenseRotationSequenceDot=off  SenseAlphaX=off  SenseAlphaY=off  SenseAlphaZ=off  SenseQDDot=off  SenseRDDot=off  SenseX=off  SenseY=on  SenseZ=on  SenseRad=off  SenseAzim=off  SenseDist=off  SenseInc=off  SenseXDot=off  SenseYDot=off  SenseZDot=off  SenseRadDot=off  SenseAzimDot=off  SenseDistDot=off  SenseIncDot=off  SenseXDDot=off  SenseYDDot=off  SenseZDDot=off  SenseRadDDot=off  SenseAzimDDot=off  SenseDistDDot=off  SenseIncDDot=off
  MATLAB Function : MATLAB Function  TreatAsAtomicUnit=on
  Multiply{,1..17} (18 alike) : Gain  Gain=1000
  PS-Simulink Converter{,6..7,11..25} (18 alike) : nesl_utility/PS-Simulink Converter  PhysicalDomain=network_engine_domain  SubClassName=ps_output  LeftPortType=input  RightPortType=output  PseudoPeriodic=off  Frequencies=[]  VectorFormat=inherit  Unit=inherit  AffineConversion=off
  Rigid Transform : sm_lib/Frames and Transforms/Rigid Transform  TranslationMethod=Cartesian  TranslationStandardOffset=0  TranslationStandardOffsetUnits=m  TranslationStandardAxis=+Z  TranslationCartesianOffset=[0 0 0]  TranslationCartesianOffsetUnits=mm  TranslationROffset=0  TranslationROffsetUnits=m  TranslationZOffset=0  TranslationZOffsetUnits=m  TranslationThetaOffset=0  TranslationThetaOffsetUnits=deg  RotationMethod=None  RotationAngleUnits=deg  RotationStandardAxis=+Z  RotationAngle=0.0  RotationArbitraryAxis=[0 0 1]  FollAlignAxisA=+X  BaseAlignAxisA=+Y  FollAlignAxisB=+Y  BaseAlignAxisB=+Z  RotationSequenceAxes=FollowerAxes  RotationSequence=XYX  RotationSequenceAngles=[0 0 0]  RotationSequenceAnglesUnits=deg  RotationMatrix=[1 0 0; 0 1 0; 0 0 1]  Quaternion=[1 0 0 0]
  S1-T1 final flexion angle : Display
  Scope4 : Scope
  T1 Position : sm_lib/Frames and Transforms/Transform Sensor  MeasurementFrame=World  RotationSequence=XYX  SenseAngle=off  SenseAxis=off  SenseQ=off  SenseR=off  SenseRotationSequence=off  SenseOmegaX=off  SenseOmegaY=off  SenseOmegaZ=off  SenseQDot=off  SenseRDot=off  SenseRotationSequenceDot=off  SenseAlphaX=off  SenseAlphaY=off  SenseAlphaZ=off  SenseQDDot=off  SenseRDDot=off  SenseX=off  SenseY=on  SenseZ=on  SenseRad=off  SenseAzim=off  SenseDist=off  SenseInc=off  SenseXDot=off  SenseYDot=off  SenseZDot=off  SenseRadDot=off  SenseAzimDot=off  SenseDistDot=off  SenseIncDot=off  SenseXDDot=off  SenseYDDot=off  SenseZDDot=off  SenseRadDDot=off  SenseAzimDDot=off  SenseDistDDot=off  SenseIncDDot=off
  T10 Position : sm_lib/Frames and Transforms/Transform Sensor  MeasurementFrame=World  RotationSequence=XYX  SenseAngle=off  SenseAxis=off  SenseQ=off  SenseR=off  SenseRotationSequence=off  SenseOmegaX=off  SenseOmegaY=off  SenseOmegaZ=off  SenseQDot=off  SenseRDot=off  SenseRotationSequenceDot=off  SenseAlphaX=off  SenseAlphaY=off  SenseAlphaZ=off  SenseQDDot=off  SenseRDDot=off  SenseX=off  SenseY=on  SenseZ=on  SenseRad=off  SenseAzim=off  SenseDist=off  SenseInc=off  SenseXDot=off  SenseYDot=off  SenseZDot=off  SenseRadDot=off  SenseAzimDot=off  SenseDistDot=off  SenseIncDot=off  SenseXDDot=off  SenseYDDot=off  SenseZDDot=off  SenseRadDDot=off  SenseAzimDDot=off  SenseDistDDot=off  SenseIncDDot=off
  T12 Position : sm_lib/Frames and Transforms/Transform Sensor  MeasurementFrame=World  RotationSequence=XYX  SenseAngle=off  SenseAxis=off  SenseQ=off  SenseR=off  SenseRotationSequence=off  SenseOmegaX=off  SenseOmegaY=off  SenseOmegaZ=off  SenseQDot=off  SenseRDot=off  SenseRotationSequenceDot=off  SenseAlphaX=off  SenseAlphaY=off  SenseAlphaZ=off  SenseQDDot=off  SenseRDDot=off  SenseX=off  SenseY=on  SenseZ=on  SenseRad=off  SenseAzim=off  SenseDist=off  SenseInc=off  SenseXDot=off  SenseYDot=off  SenseZDot=off  SenseRadDot=off  SenseAzimDot=off  SenseDistDot=off  SenseIncDot=off  SenseXDDot=off  SenseYDDot=off  SenseZDDot=off  SenseRadDDot=off  SenseAzimDDot=off  SenseDistDDot=off  SenseIncDDot=off
  T5 Position : sm_lib/Frames and Transforms/Transform Sensor  MeasurementFrame=World  RotationSequence=XYX  SenseAngle=off  SenseAxis=off  SenseQ=off  SenseR=off  SenseRotationSequence=off  SenseOmegaX=off  SenseOmegaY=off  SenseOmegaZ=off  SenseQDot=off  SenseRDot=off  SenseRotationSequenceDot=off  SenseAlphaX=off  SenseAlphaY=off  SenseAlphaZ=off  SenseQDDot=off  SenseRDDot=off  SenseX=off  SenseY=on  SenseZ=on  SenseRad=off  SenseAzim=off  SenseDist=off  SenseInc=off  SenseXDot=off  SenseYDot=off  SenseZDot=off  SenseRadDot=off  SenseAzimDot=off  SenseDistDot=off  SenseIncDot=off  SenseXDDot=off  SenseYDDot=off  SenseZDDot=off  SenseRadDDot=off  SenseAzimDDot=off  SenseDistDDot=off  SenseIncDDot=off
  Conn1 : PMIOPort  Side=Right
  Conn2 : PMIOPort  Port=2  Side=Right
  Conn3 : PMIOPort  Port=3  Side=Right
  Conn4 : PMIOPort  Port=4  Side=Right
  Conn5 : PMIOPort  Port=5  Side=Left
  Conn6 : PMIOPort  Port=6  Side=Right
  Conn7 : PMIOPort  Port=7  Side=Right
  Conn8 : PMIOPort  Port=8  Side=Right
  Conn9 : PMIOPort  Port=9  Side=Right
  Conn10 : PMIOPort  Port=10  Side=Right
  wires:
  PS-Simulink Converter6/1 -> MATLAB Function/2(z), Multiply1/1
  PS-Simulink Converter16/1 -> Multiply10/1
  Multiply4/1 -> Display5/1
  Multiply3/1 -> Display4/1
  PS-Simulink Converter/1 -> Multiply/1, MATLAB Function/1(y)
  Multiply1/1 -> Display2/1
  PS-Simulink Converter17/1 -> Multiply11/1
  PS-Simulink Converter22/1 -> Multiply15/1
  PS-Simulink Converter14/1 -> Multiply2/1
  Multiply9/1 -> Display10/1
  PS-Simulink Converter15/1 -> Multiply3/1
  PS-Simulink Converter19/1 -> Multiply7/1
  PS-Simulink Converter20/1 -> Multiply13/1
  Multiply13/1 -> Display13/1
  Multiply10/1 -> Display11/1
  Multiply12/1 -> Display14/1
  MATLAB Function/1(angle) -> S1-T1 final flexion angle/1, Scope4/1
  PS-Simulink Converter18/1 -> Multiply6/1
  PS-Simulink Converter23/1 -> Multiply14/1
  PS-Simulink Converter7/1 -> Multiply8/1
  Multiply2/1 -> Display3/1
  Multiply7/1 -> Display8/1
  Multiply/1 -> Display1/1
  Multiply5/1 -> Display6/1
  Multiply6/1 -> Display7/1
  PS-Simulink Converter11/1 -> Multiply9/1
  Multiply11/1 -> Display12/1
  PS-Simulink Converter13/1 -> Multiply5/1
  Multiply16/1 -> Display18/1
  PS-Simulink Converter12/1 -> Multiply4/1
  Multiply14/1 -> Display16/1
  PS-Simulink Converter21/1 -> Multiply12/1
  Multiply8/1 -> Display9/1
  Multiply15/1 -> Display15/1
  PS-Simulink Converter25/1 -> Multiply16/1
  Multiply17/1 -> Display17/1
  PS-Simulink Converter24/1 -> Multiply17/1
  connections:
  T1 Position/LConn1 -- T12 Position/LConn1 -- L1 Spinous Process Position/LConn1 -- L2 Spinous process Position/LConn1 -- L3 Spinous process Position/LConn1 -- L5 Spinous Process Position/LConn1 -- Rigid Transform/RConn1 -- L4 Spinous Process Position/LConn1 -- T10 Position/LConn1 -- T5 Position/LConn1
  T1 Position/RConn2 -- PS-Simulink Converter/LConn1
  T12 Position/RConn3 -- PS-Simulink Converter24/LConn1
  Conn3/RConn1 -- L1 Spinous Process Position/RConn1
  L2 Spinous process Position/RConn2 -- PS-Simulink Converter16/LConn1
  L5 Spinous Process Position/RConn2 -- PS-Simulink Converter7/LConn1
  L4 Spinous Process Position/RConn3 -- PS-Simulink Converter13/LConn1
  T1 Position/RConn1 -- Conn8/RConn1
  L3 Spinous process Position/RConn1 -- Conn2/RConn1
  Conn1/RConn1 -- L2 Spinous process Position/RConn1
  L2 Spinous process Position/RConn3 -- PS-Simulink Converter17/LConn1
  T12 Position/RConn2 -- PS-Simulink Converter25/LConn1
  T10 Position/RConn3 -- PS-Simulink Converter22/LConn1
  L1 Spinous Process Position/RConn3 -- PS-Simulink Converter19/LConn1
  L5 Spinous Process Position/RConn1 -- Conn6/RConn1
  L4 Spinous Process Position/RConn2 -- PS-Simulink Converter12/LConn1
  T10 Position/RConn2 -- PS-Simulink Converter23/LConn1
  T1 Position/RConn3 -- PS-Simulink Converter6/LConn1
  Rigid Transform/LConn1 -- Conn5/RConn1
  L3 Spinous process Position/RConn2 -- PS-Simulink Converter14/LConn1
  PS-Simulink Converter21/LConn1 -- T5 Position/RConn2
  T12 Position/RConn1 -- Conn10/RConn1
  L1 Spinous Process Position/RConn2 -- PS-Simulink Converter18/LConn1
  L5 Spinous Process Position/RConn3 -- PS-Simulink Converter11/LConn1
  L3 Spinous process Position/RConn3 -- PS-Simulink Converter15/LConn1
  PS-Simulink Converter20/LConn1 -- T5 Position/RConn3
  L4 Spinous Process Position/RConn1 -- Conn4/RConn1
  T5 Position/RConn1 -- Conn7/RConn1
  T10 Position/RConn1 -- Conn9/RConn1
